simulink model "dspintrpf"  (Simulink 6.0)
settings: Solver=FixedStepDiscrete  SolverMode=SingleTasking  StartTime=0.0  StopTime=50.0  RelTol=1e-3  AbsTol=1e-6
undefined symbols (not defined in the file or in its folder): intfilt
libraries: dspbuff3 x2, dspsigops x1, dspmlti3 x1, dspsrcs4 x1
settings Model: CovMetricSettings=d  Creator=don  LastModifiedBy=sconahan  ExtModeTrigMode=oneshot  ExtModeArmWhenConnect=off
settings DataIOCC: LimitDataPoints=off  SaveOutput=off  SaveTime=off  SignalLoggingName=sigsOut
settings OptimizationCC: BlockReduction=off  BooleanDataType=off  MultiInstanced=off  RollThreshold=2
settings FormatCC: IgnoreBidirectionalLines=off
settings DebuggingCC: SingleTaskRateTransMsg=error  IntegerOverflowMsg=none
settings HardwareCC: TargetUnknown=on
settings CodeAppCC: FileBanners=off  CustomSymbols=off
settings GRTTargetCC: TargetFcnLib=iso_c_tmw.mat  IsERTTarget=off

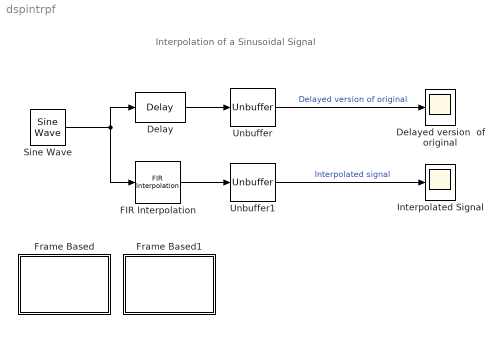
== system dspintrpf ==
  note: Interpolation of a Sinusoidal Signal
  Delay : dspsigops/Delay  dly_unit=Samples  delay=9  ic_detail=on  dif_ic_for_ch=off  dif_ic_for_dly=off  ic=0  reset_popup=None
  Delayed version  of original : Scope
      settings: TickLabels=on  YMin=-1.2  YMax=1.2  DataFormat=Array
  FIR Interpolation : dspmlti3/FIR Interpolation  h=intfilt(9, 9, .5)  L=9  framing=Maintain input frame size  outputBufInitCond=0  roundingMode=Floor  overflowMode=off
  Frame Based : Subsystem
      settings: OpenFcn=dspintrp
      mask Display: disp('Sample-based\nVersion')
  Frame Based1 : Subsystem
      settings: OpenFcn=dspintrpfp
      mask Display: disp('Fixed-point\nVersion')
  Interpolated Signal : Scope
      settings: TickLabels=on  YMin=-1.2  YMax=1.2  DataFormat=Array
  Sine Wave : dspsrcs4/Sine Wave  Amplitude=1  Frequency=0.2  Phase=0.7  SampleMode=Discrete  OutComplex=Real  CompMethod=Trigonometric fcn  TableSize=Speed  SampleTime=1  SamplesPerFrame=32  dataType=double  wordLen=16  udDataType=sfix(16)  fracBitsMode=Best precision  numFracBits=15  ResetState=Restart at time zero
  Unbuffer : dspbuff3/Unbuffer  ic=0
  Unbuffer1 : dspbuff3/Unbuffer  ic=0
  wires:
  Sine Wave/1 -> FIR Interpolation/1, Delay/1
  Delay/1 -> Unbuffer/1
  Unbuffer/1 -> Delayed version  of original/1  "Delayed version of original"
  FIR Interpolation/1 -> Unbuffer1/1
  Unbuffer1/1 -> Interpolated Signal/1  "Interpolated signal"

== system dspintrpf/Frame Based ==

== system dspintrpf/Frame Based1 ==
